simulink model "FactorialFlowChart"  (R2018b)
settings: Solver=VariableStepAuto  StartTime=0.0  StopTime=10.0  RelTol=1e-3
settings Model: Creator=Ahmed Soliman  LastModifiedBy=Ahmed Soliman

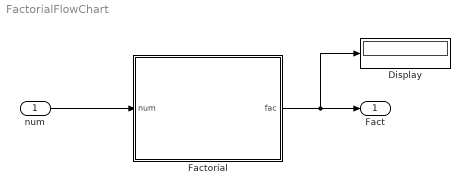
== system FactorialFlowChart ==
  "num " : Inport  OutDataTypeStr=uint16
  Display : Display
  Factorial : Stateflow chart  TreatAsAtomicUnit=on
  Fact : Outport  OutDataTypeStr=uint32
  wires:
  "num "/1 -> Factorial/1(num)
  Factorial/1(fac) -> Fact/1, Display/1

== stateflow chart FactorialFlowChart/Factorial ==
  (default) -> (junction 10) : /* Factorial */
  (junction 11) -> (junction 6) [order 1] : [i > 0]
  (junction 6) -> (junction 8) : {fac=fac*i;}
  (junction 10) -> (junction 11) : {i = num;fac=1}
  (junction 8) -> (junction 11) : {i--;}
  (junction 11) -> (junction 9) [order 2]
  data: fac output uint32; num input uint16; i local uint16
